simulink model "open_loop"  (R2022b)
settings: Solver=FixedStepAuto  StartTime=0.0  StopTime=20  FixedStep=1/100  RelTol=1e-3  AbsTol=1e-3
model workspace: external: MATLAB File params.m (data not in the file)
values from neighbouring files (symbols this model uses):
  drag = 2.5383e-11    [Linearization.m]    (also in params.m)
  g = 9.81    [Linearization.m]    (also in params.m)
  lift = 1.9796e-9    (= 1.9796e-09)    [Linearization.m]    (also in params.m)
  m = 0.027    [Linearization.m]    (also in params.m)
libraries: nesl_utility x9
settings Model: Creator=Jocke  LastModifiedBy=gui00
settings SolverCC: AutoScaleAbsTol=off  AlgebraicLoopSolver=TrustRegion
settings DataIOCC: ReturnWorkspaceOutputs=off
settings DebuggingCC: UnconnectedInputMsg=warning  UnconnectedOutputMsg=warning  UnconnectedLineMsg=warning  SFMachineParentedDataDiag=warning  ArithmeticOperatorsInVariantConditions=warning
settings ModelReferenceCC: EnableRefExpFcnMdlSchedulingChecks=on
settings SFSimCC: SimUseLocalCustomCode=off  CustomCodeUndefinedFunction=UseInterfaceOnly
settings RTWCC: RTWUseLocalCustomCode=off
settings CodeAppCC: StateflowObjectComments=on
settings SimscapeCC: SimscapeNormalizeSystem=off  SimscapeLogType=all  SimscapeLogDataHistory=10000

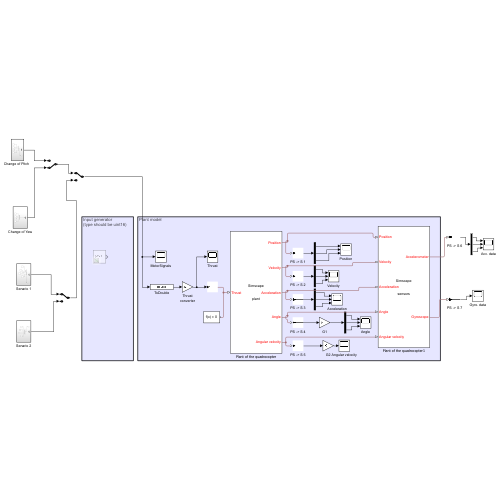
[thumbnail: Simulink's stored preview of the top-level diagram]
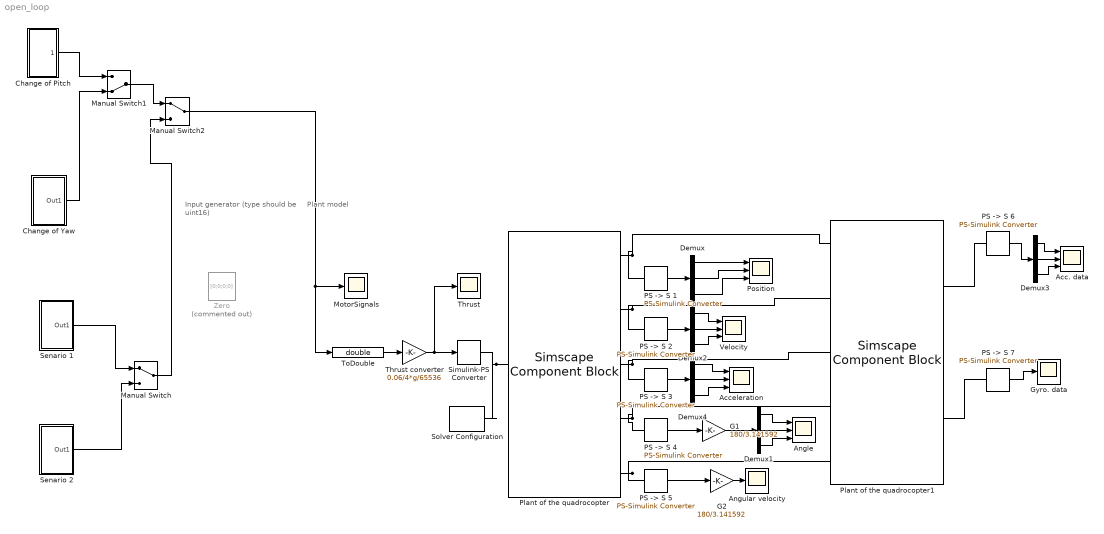
== system open_loop ==
  note: Input generator
      | (type should be uint16)
  note: Plant model
  Acc. data : Scope  NumInputPorts=3
  Acceleration : Scope  NumInputPorts=3
  Angle : Scope  NumInputPorts=3
  Angular velocity : Scope
  "Change of Pitch  " : Subsystem
  Change of Yaw : Subsystem
  Demux{,1..4} (5 alike) : Demux  Outputs=3
  G1 : Gain  Gain=180/3.141592
  G2 : Gain  Gain=180/3.141592
  Gyro. data : Scope
  Manual Switch : ManualSwitch
  Manual Switch1 : ManualSwitch  CurrentSetting=0
  Manual Switch2 : ManualSwitch
  MotorSignals : Scope
  PS -> S {1..7} (7 alike) : nesl_utility/PS-Simulink Converter  PhysicalDomain=network_engine_domain  SubClassName=ps_output  LeftPortType=input  RightPortType=output  PseudoPeriodic=off  Frequencies=[]  VectorFormat=1-D array  Unit=1  AffineConversion=off
  Plant of the quadrocopter : SimscapeComponentBlock  SourceFile=plant  ComponentPath=plant  ComponentVariants=plant  ComponentVariantNames=plant  ClassName=plant  SchemaVersion=1  m=m kg  g=g m/s^2  d=d m  lift=1.9796e-9 N*s^2/rad^2  drag=2.5383e-11 N*m*s^2/rad^2  F=0.25 N*s/m  c=0 m/s^2
      settings: CopyFcn=simscape.engine.sli.internal.componentblockcallback(gcbh,'COPY')  PreCopyFcn=simscape.engine.sli.internal.componentblockcallback(gcbh,'PRECOPY')  PreDeleteFcn=simscape.engine.sli.internal.componentblockcallback(gcbh,'PREDELETE')  InternalSimscapePortConfiguration="{\"Bottom\":[],\"Left\":[{\"id\":\"ctrl\",\"label\":\"Thrust\",\"type\":\"input\"}],\"Right\":[{\"id\":\"pos\",\"label\":\"Position\",\"type\":\"output\"},{\"id\":\"v\",\"label\":\"Velocity\",\"type\":\"output\"},{\"id\":\"a\",\"label\":\"Acceleration\",\"type\":\"output\"},{\"id\":\"angle\",\"label\":\"Angle\",\"type\":\"output\"},{\"id\":\"w\",\"label\":\"Angular velocity\",\"type\":\"output\"}],\"Top\":[]}"
      mask Type: Plant of quadrocopter
  Plant of the quadrocopter1 : SimscapeComponentBlock  SourceFile=sensors  ComponentPath=sensors  ComponentVariants=sensors  ComponentVariantNames=sensors  ClassName=sensors  SchemaVersion=1  m=m kg  g=g m/s^2  d=d m  k=drag km  b=lift
      settings: CopyFcn=simscape.engine.sli.internal.componentblockcallback(gcbh,'COPY')  PreCopyFcn=simscape.engine.sli.internal.componentblockcallback(gcbh,'PRECOPY')  PreDeleteFcn=simscape.engine.sli.internal.componentblockcallback(gcbh,'PREDELETE')  InternalSimscapePortConfiguration="{\"Bottom\":[],\"Left\":[{\"id\":\"pos\",\"label\":\"Position\",\"type\":\"input\"},{\"id\":\"v\",\"label\":\"Velocity\",\"type\":\"input\"},{\"id\":\"a\",\"label\":\"Acceleration\",\"type\":\"input\"},{\"id\":\"angle\",\"label\":\"Angle\",\"type\":\"input\"},{\"id\":\"w\",\"label\":\"Angular velocity\",\"type\":\"input\"}],\"Right\":[{\"id\":\"acc\",\"label\":\"Accelerometer\",\"type\":\"output\"},{\"id\":\"gyro\",\"label\":\"Gyroscope\",\"type\":\"output\"}],\"Top\":[]}"
      mask Type: Plant of quadrocopter
  Position : Scope  NumInputPorts=3
  Senario 1 : Subsystem
  Senario 2 : Subsystem
  Simulink-PS Converter : nesl_utility/Simulink-PS Converter  PhysicalDomain=network_engine_domain  SubClassName=ps_input  LeftPortType=input  RightPortType=output  PseudoPeriodic=off  Frequencies=[]  NoiseDistribution=none  NoiseParameters=[]  Unit=1  AffineConversion=off  FilteringAndDerivatives=zero  SimscapeFilterOrder=1  InputFilterTimeConstant=0.001  UdotUserProvided=1
  Solver Configuration : nesl_utility/Solver Configuration  PhysicalDomain=network_engine_domain  SubClassName=solver  LeftPortType=input  RightPortType=generic  Tones=[]  Harmonics=[]  SimulateNoise=off  Profile=off  UseLocalSampling=off  EnableSwitchedLinearOptims=on  FrequencyDomain=off  UseCCode=off  RelTol=0.001  AbsTol=1e-06  MinStep=1e-09  ToWorkspace=off  RevertToSquareIcSolve=off  NumHomotopyIterations=100  PhasorMode=off  PhasorModeNumHarmonics=1  ConsistencySolver=NEWTON_FTOL  IndexReductionMethod=DerivativeReplacement  DoDC=off  ResidualTolerance=1e-09  ConsistencyTolSource=GLOBAL  ConsistencyAbsTol=0.001  ConsistencyRelTol=0.001  ConsistencyTolFactor=0.001  UseLocalSolver=off  LocalSolverChoice=NE_BACKWARD_EULER_ADVANCER  ResolveIndetEquations=on  FunctionEvalNumThread=1  LocalSolverSampleTime=0.001  DoFixedCost=off  MaxNonlinIter=3  MaxModeIter=2  ComputeImpulses=off  ImpulseIterations=2  LinearAlgebra=Sparse  LinearAlgebraNumThread=0  EquationFormulation=NE_TIME_EF  DelaysMemoryBudget=1024  AutomaticFiltering=on  FilteringTimeConstant=0.001  PartitionStorageMethod=AS_NEEDED  PartitionMemoryBudget=1024  PartitionMethod=FAST
  Thrust : Scope
  Thrust converter : Gain  Gain=0.06/4*g/65536
  ToDouble : DataTypeConversion  OutDataTypeStr=double  RndMeth=Round
  Velocity : Scope  NumInputPorts=3
  Zero : Constant  Commented=on  Value=[0;0;0;0]  VectorParams1D=off  OutDataTypeStr=uint16
  wires:
  "PS -> S 7"/1 -> Gyro. data/1
  G2/1 -> Angular velocity/1
  ToDouble/1 -> Thrust converter/1
  Thrust converter/1 -> Thrust/1, Simulink-PS Converter/1
  "PS -> S 5"/1 -> G2/1
  "PS -> S 4"/1 -> G1/1
  "PS -> S 1"/1 -> Demux/1
  Demux/1 -> Position/1
  Demux/2 -> Position/2
  Demux/3 -> Position/3
  Manual Switch/1 -> Manual Switch2/2
  G1/1 -> Demux1/1
  Demux1/1 -> Angle/1
  Demux1/2 -> Angle/2
  Demux1/3 -> Angle/3
  Manual Switch1/1 -> Manual Switch2/1
  Manual Switch2/1 -> ToDouble/1, MotorSignals/1
  "PS -> S 2"/1 -> Demux2/1
  Demux2/3 -> Velocity/3
  Demux2/2 -> Velocity/2
  Demux2/1 -> Velocity/1
  "PS -> S 6"/1 -> Demux3/1
  Demux3/1 -> Acc. data/1
  Demux3/2 -> Acc. data/2
  Demux3/3 -> Acc. data/3
  Demux4/3 -> Acceleration/3
  Demux4/2 -> Acceleration/2
  Demux4/1 -> Acceleration/1
  "PS -> S 3"/1 -> Demux4/1
  Senario 1/1(Out1) -> Manual Switch/1
  Senario 2/1(Out1) -> Manual Switch/2
  Change of Yaw/1(Out1) -> Manual Switch1/2
  "Change of Pitch  "/1(Out1) -> Manual Switch1/1
  connections:
  Plant of the quadrocopter/LConn1 -- Simulink-PS Converter/RConn1 -- Solver Configuration/RConn1
  Plant of the quadrocopter/RConn1 -- "PS -> S 1"/LConn1 -- Plant of the quadrocopter1/LConn1
  Plant of the quadrocopter/RConn2 -- "PS -> S 2"/LConn1 -- Plant of the quadrocopter1/LConn2
  Plant of the quadrocopter/RConn3 -- Plant of the quadrocopter1/LConn3 -- "PS -> S 3"/LConn1
  Plant of the quadrocopter/RConn4 -- Plant of the quadrocopter1/LConn4 -- "PS -> S 4"/LConn1
  Plant of the quadrocopter/RConn5 -- Plant of the quadrocopter1/LConn5 -- "PS -> S 5"/LConn1
  "PS -> S 6"/LConn1 -- Plant of the quadrocopter1/RConn1
  Plant of the quadrocopter1/RConn2 -- "PS -> S 7"/LConn1

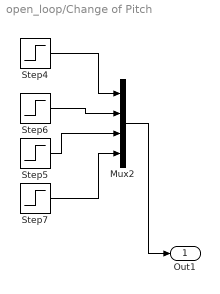
== system open_loop/Change of Pitch   ==
  Mux2 : Mux
  Step4 : Step  Time=5  After=1000  SampleTime=0
  Step5 : Step  Time=5  Before=1000  After=0  SampleTime=0
  Step6 : Step  Time=5  Before=1000  After=0  SampleTime=0
  Step7 : Step  Time=5  After=1000  SampleTime=0
  Out1 : Outport
  wires:
  Step4/1 -> Mux2/1
  Step6/1 -> Mux2/2
  Mux2/1 -> Out1/1
  Step7/1 -> Mux2/4
  Step5/1 -> Mux2/3

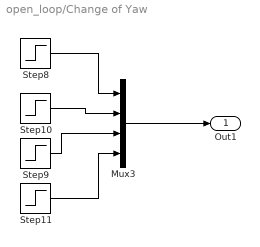
== system open_loop/Change of Yaw ==
  Mux3 : Mux
  Step10 : Step  Time=5  Before=1000  After=0  SampleTime=0
  Step11 : Step  Time=5  Before=1000  After=0  SampleTime=0
  Step8 : Step  Time=5  After=1000  SampleTime=0
  Step9 : Step  Time=5  After=1000  SampleTime=0
  Out1 : Outport
  wires:
  Step10/1 -> Mux3/2
  Step9/1 -> Mux3/3
  Mux3/1 -> Out1/1
  Step11/1 -> Mux3/4
  Step8/1 -> Mux3/1

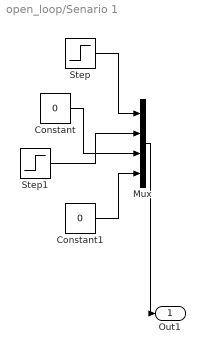
== system open_loop/Senario 1 ==
  Constant : Constant  Value=0
  Constant1 : Constant  Value=0
  Mux : Mux
  Step : Step  Time=4  After=10  SampleTime=0
  Step1 : Step  Time=4  After=10  SampleTime=0
  Out1 : Outport
  wires:
  Constant1/1 -> Mux/4
  Constant/1 -> Mux/3
  Step/1 -> Mux/1
  Step1/1 -> Mux/2
  Mux/1 -> Out1/1

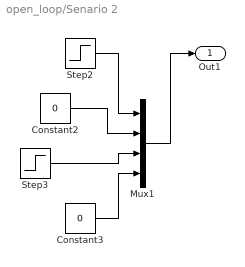
== system open_loop/Senario 2 ==
  Constant2 : Constant  Value=0
  Constant3 : Constant  Value=0
  Mux1 : Mux
  Step2 : Step  Time=4  After=1000  SampleTime=0
  Step3 : Step  Time=6  After=2000  SampleTime=0
  Out1 : Outport
  wires:
  Constant2/1 -> Mux1/2
  Constant3/1 -> Mux1/4
  Step2/1 -> Mux1/1
  Step3/1 -> Mux1/3
  Mux1/1 -> Out1/1
